simulink model "test"  (R2015a)
settings: Solver=ode45  StartTime=0.0  StopTime=10.0  RelTol=1e-3
settings Model: Creator=shohei  LastModifiedBy=shohei

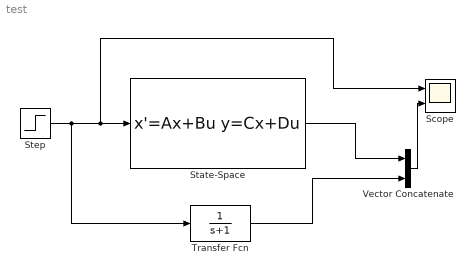
== system test ==
  Scope : Scope  NumInputPorts=2
      settings: YMin=-5~-5  YMax=5~5
  State-Space : StateSpace  A=-1  D=0  X0=0
  Step : Step  SampleTime=0
  Transfer Fcn : TransferFcn  Denominator=[1 1]
  Vector Concatenate : Concatenate
  wires:
  Step/1 -> Transfer Fcn/1, Scope/1, State-Space/1
  State-Space/1 -> Vector Concatenate/1
  Transfer Fcn/1 -> Vector Concatenate/2
  Vector Concatenate/1 -> Scope/2
